simulink model "Core_Communication_System_Model"  (R2022b)
settings: Solver=VariableStepAuto  StartTime=0.0  StopTime=10  RelTol=1e-3
values from neighbouring files (symbols this model uses):
  Bit_period = (1/Sampling_rate)/(Quantization)    (= 6.25e-06)    [Model_Paramters.m]
  Filter_span = 4    [Model_Paramters.m]
  Ns = 400    [Model_Paramters.m]
  Roll_off = 0.8    [Model_Paramters.m]
  Sampling_rate = 10000    [Model_Paramters.m]
libraries: commdigbbndpm3 x2, simulink x2, dspvision x2, commblkcod2 x2, commfilt2 x2, commchan3 x1, commsink2 x1
settings Model: Creator=Aman  LastModifiedBy=Aman

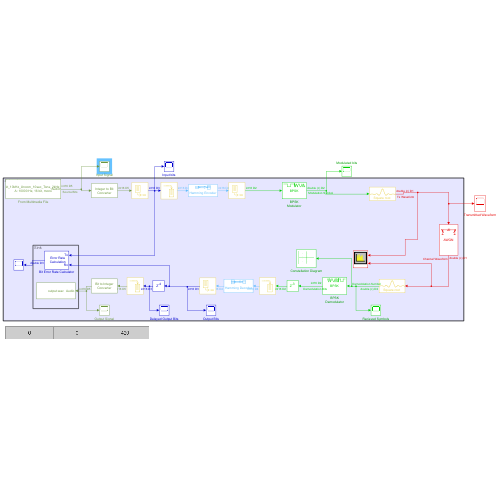
[thumbnail: Simulink's stored preview of the top-level diagram]
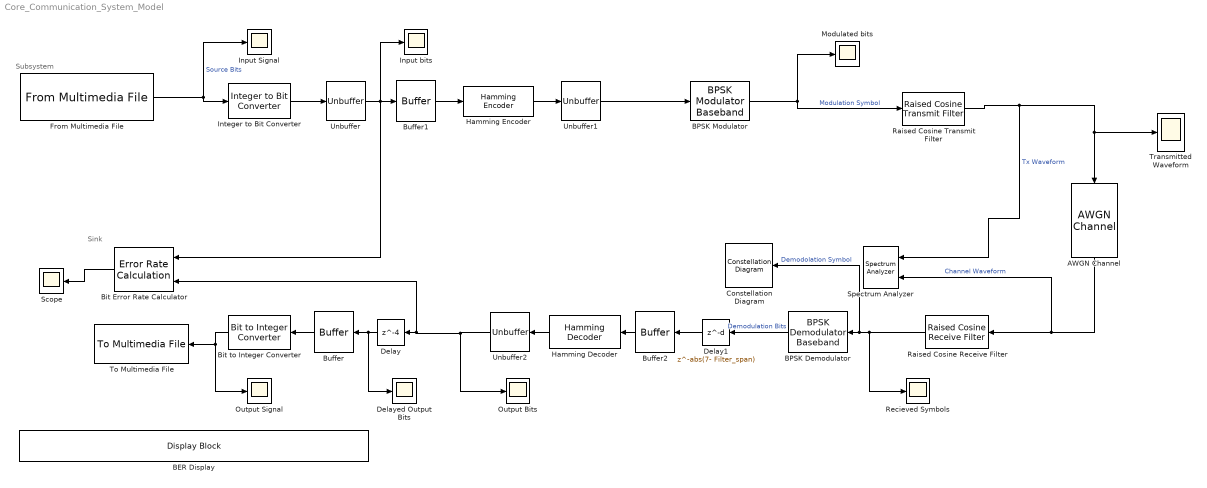
== system Core_Communication_System_Model ==
  note: Sink
  note: Subsystem
  AWGN Channel : commchan3/AWGN Channel  InputProcessing=Columns as channels (frame based)  seed=RandomSeed  noiseMode="Signal to noise ratio  (Eb/No)"  EbNodB=SNR  EsNodB=SNR  SNRdB=SNR  bitsPerSym=1  Ps=1  Tsym=Bit_period/Ns  variance=0.4
  BER Display : DisplayBlock  LabelPosition=Hide  Transparency=1
  "BPSK Demodulator " : commdigbbndpm3/BPSK Demodulator Baseband  DecType=Hard decision  VarSource=Dialog  Variance=0.4  Ph=0  outDtype=int16  derotateFactorWordLen=16  derotateFactorDataTypeStr=Inherit: Same word length as input  derotateFactorLastDataTypeStr=Inherit: Same word length as input
  "BPSK Modulator " : commdigbbndpm3/BPSK Modulator Baseband  Ph=0  outDtype=double  outWordLen=16  outUDDataType=sfix(16)  outFracLenMode=Best precision  outFracLen=15  outDataTypeStr=double  outLastDataTypeStr=double
  Bit Error Rate Calculator : commsink2/Error Rate Calculation  N=12  st_delay=0  cp_mode=Entire frame  subframe=[]  PMode=Port  WsName=ErrorVec  RsMode2=off  stop=on  numErr=MaxErrors  maxBits=MaxBits
  Bit to Integer Converter : simulink/Logic and Bit Operations/Bit to Integer Converter  nbits=16  bitOrder=MSB first  signedOutputValues=Signed  outDtype=int16  outDtypeSigned=int16
  Buffer : Buffer  N=16  OutputFrames=off
  Buffer1 : Buffer  N=4  OutputFrames=off
  Buffer2 : Buffer  N=7  OutputFrames=off
  Constellation Diagram : ConstellationDiagram  WindowPosition=[382.000000,84.000000,600.000000,600.000000,]  ScopeFrameLocation=window  SymbolsToDisplaySource=Property  SymbolsToDisplay=MaxBits  ReferenceConstellation=BPSK  XLimits=[-1.46,1.46]  YLimits=[-1.38,1.38]
  Delay : Delay  DelayLength=4  InitialCondition=0
  Delay1 : Delay  DelayLength=abs(7- Filter_span)  InitialCondition=0
  Delayed Output Bits : Scope
  From Multimedia File : dspvision/From Multimedia File  inputFilename=C:\Users\Aman\Desktop\ELEC-391\ELEC391_Sound_Files\Mono_16bit_10kHz_Uncom_10sec_Tone_2kHz_4kHz.wav  readRange=[1 5000]  loop=on  numPlays=1  outputStreams=Audio only  videoDataType=single  audioDataType=int16  inheritSampleTime=off  userDefinedSampleTime=1/Sampling_rate  noAudioOutput=off  isIntensityVideo=off  fourcc=RGB  colorVideoFormat=Separate color signals  outputEOF=off  dataOrg=Column-major  audioFrameSize=1  computeAudioFrameSize=off  outSamplingMode=Sample based
      settings: LibrarySourceBlock=dspsrcs4/From Multimedia File
  Hamming Decoder : commblkcod2/Hamming Decoder  n=7  k=4
  Hamming Encoder : commblkcod2/Hamming Encoder  n=7  k=4
  Input Signal : Scope
  Input bits : Scope
  Integer to Bit Converter : simulink/Logic and Bit Operations/Integer to Bit Converter  nbits=Quantization  signedInputValues=Signed  bitOrder=MSB first  outDtype=int16
  Modulated bits : Scope
  Output Bits : Scope
  Output Signal : Scope
  Raised Cosine Receive Filter : commfilt2/Raised Cosine Receive Filter  filtType=Square root  R=Roll_off  filtSpan=Filter_span  N=Ns  downFactor=Ns  downOffset=0  filterGain=1  RateOptions=Allow multirate processing  framing=Mute  checkCoeff=off  variableName=rcRxFilt  currentFiltSpan=10  D=5  inputOffset=0  sampMode=Mute  saveAsFlag=0  rateMode=Downsampling  checkGain=Normalized  launchFVT=on  roundingMode=Floor  overflowMode=off  coeffDataTypeStr=Inherit: Same word length as input  coeffMin=[]  coeffMax=[]  coeffLastDataTypeStr=Inherit: Same word length as input  accumDataTypeStr=Inherit: Same as product output  accumLastDataTypeStr=Inherit: Same as product output  outputDataTypeStr=Inherit: Same as accumulator  outputMin=[]  outputMax=[]  outputLastDataTypeStr=Inherit: Same as accumulator
  Raised Cosine Transmit Filter : commfilt2/Raised Cosine Transmit Filter  filtType=Square root  R=Roll_off  filtSpan=Filter_span  N=Ns  filterGain=1  RateOptions=Allow multirate processing  framing=Mute  checkCoeff=on  variableName=exported_filter_coeffs  checkGain=Normalized  sampMode=Mute  saveAsFlag=0  currentFiltSpan=10  D=(10)/2  launchFVT=on  roundingMode=Floor  overflowMode=off  coeffDataTypeStr=Inherit: Same word length as input  coeffMin=[]  coeffMax=[]  coeffLastDataTypeStr=Inherit: Same word length as input  outputDataTypeStr=Inherit: Same as accumulator  outputMin=[]  outputMax=[]  outputLastDataTypeStr=Inherit: Same as accumulator
  Recieved Symbols : Scope
  Scope : Scope
  Spectrum Analyzer : SpectrumAnalyzer  NumInputPorts=2
  To Multimedia File : dspvision/To Multimedia File  outputFilename=output.wav  streamSelection=Audio only  videoCompressor=None (uncompressed)  audioCompressor=None (uncompressed)  imagePorts=Separate color signals  fileType=WAV  audioDatatype=16-bit integer  fourcc=RGB  videoQuality=75  mj2000CompFactor=10
      settings: LibrarySourceBlock=dspsnks4/To Multimedia File
  Transmitted Waveform : Scope
  Unbuffer : Unbuffer
  Unbuffer1 : Unbuffer
  Unbuffer2 : Unbuffer
  wires:
  Bit Error Rate Calculator/1 -> Scope/1
  Raised Cosine Transmit Filter/1 -> AWGN Channel/1, Transmitted Waveform/1, Spectrum Analyzer/1  "Tx Waveform"
  "BPSK Modulator "/1 -> Raised Cosine Transmit Filter/1, Modulated bits/1  "Modulation Symbol"
  From Multimedia File/1 -> Integer to Bit Converter/1, Input Signal/1  "Source Bits"
  "BPSK Demodulator "/1 -> Delay1/1  "Demodulation Bits"
  AWGN Channel/1 -> Raised Cosine Receive Filter/1, Spectrum Analyzer/2  "Channel Waveform"
  Raised Cosine Receive Filter/1 -> Constellation Diagram/1, "BPSK Demodulator "/1, Recieved Symbols/1  "Demodolation Symbol"
  Integer to Bit Converter/1 -> Unbuffer/1
  Unbuffer/1 -> Input bits/1, Bit Error Rate Calculator/1, Buffer1/1
  Buffer/1 -> Bit to Integer Converter/1
  Bit to Integer Converter/1 -> Output Signal/1, To Multimedia File/1
  Delay/1 -> Delayed Output Bits/1, Buffer/1
  Buffer1/1 -> Hamming Encoder/1
  Hamming Encoder/1 -> Unbuffer1/1
  Unbuffer1/1 -> "BPSK Modulator "/1
  Hamming Decoder/1 -> Unbuffer2/1
  Buffer2/1 -> Hamming Decoder/1
  Unbuffer2/1 -> Output Bits/1, Bit Error Rate Calculator/2, Delay/1
  Delay1/1 -> Buffer2/1
